simulink model "Commercial_Power_Generation_and_Transmission"  (R2022b)
settings: Solver=VariableStepAuto  StartTime=0.0  StopTime=10.0  RelTol=1e-3
libraries: spsExcitationSystemLib x6, spsHydraulicTurbineandGovernorLib x6, spsSynchronousMachinepuFundamentalLib x6, spsThreePhaseTransformerTwoWindingsLib x4, spsLoadFlowBusLib x2, spsThreePhaseParallelRLCLoadLib x2, spsGroundLib x1, spsThreePhaseFaultLib x1, spsThreePhaseSourceLib x1, spsVoltageMeasurementLib x1, spspowerguiLib x1
settings Model: Creator=admin  LastModifiedBy=USER
settings SolverCC: AlgebraicLoopSolver=TrustRegion
settings DebuggingCC: UnconnectedInputMsg=warning  UnconnectedOutputMsg=warning  UnconnectedLineMsg=warning
settings ModelReferenceCC: EnableRefExpFcnMdlSchedulingChecks=on
settings RTWCC: GenCodeOnly=on

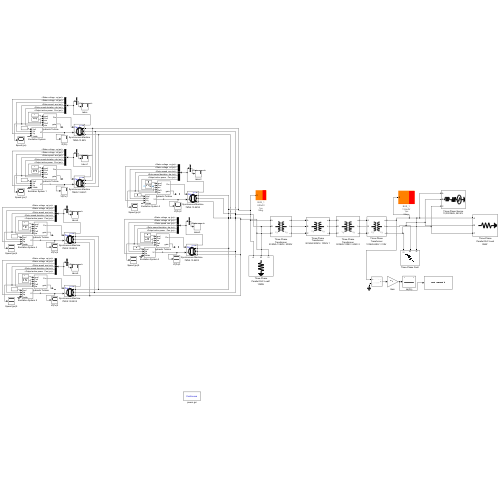
[thumbnail: Simulink's stored preview of the top-level diagram]
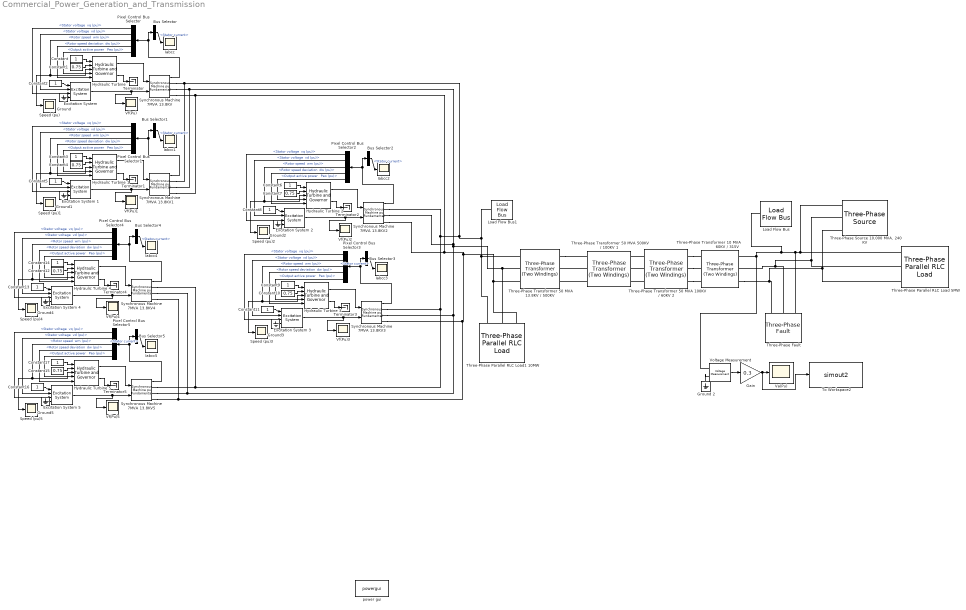
== system Commercial_Power_Generation_and_Transmission ==
  Bus Selector{,1..5} (6 alike) : BusSelector  OutputSignals=Stator current
  Constant{,2..3,5..6,8..9,11,13..14,16..17} (12 alike) : Constant
  Constant{1,4,7,10,12,15} (6 alike) : Constant  Value=0.75
  Excitation System {,1..5} (6 alike) : spsExcitationSystemLib/Excitation System  tr=20e-3  reg=[ 300, 0.001 ]  exc=[ 1, 0 ]  tgr=[ 0, 0 ]  damp=[ 0.001, 0.1 ]  sat=[ 0, 0 ]  lim=[ -11.5, 11.5, 0 ]  v0="[1.0  1.28]"
  "Gain " : Gain  Gain=0.3
  Ground{,1..5} (6 alike) : Ground
  "Ground 2 " : spsGroundLib/Ground  LConnTagsString=a
  Hydraulic Turbine {,1..5} (6 alike) : spsHydraulicTurbineandGovernorLib/Hydraulic Turbine and Governor  sm="[ 10/3  0.07 ]"  gate="[  0.01  0.97518  -0.1  0.1 ]"  reg="[  0.05  1.163  0.105  0  0.01  ]"  hyd="[  0  2.67  ]"  dref=0  po=0.7516
  Iabcc{,1..5} (6 alike) : Scope
  Load Flow Bus : spsLoadFlowBusLib/Load Flow Bus  LConnTagsString=a  Phases=single  Connectors=on one side  ID=BUS_1  Vbase=13.8e3  Vref=1  Vangle=0  VLF=1  VLFb=1  VLFc=1  angleLF=0  angleLFb=0  angleLFc=0
  Load Flow Bus1 : spsLoadFlowBusLib/Load Flow Bus  LConnTagsString=a  Phases=single  Connectors=on one side  ID=BUS_1  Vbase=240e3  Vref=1  Vangle=0  VLF=1  VLFb=1  VLFc=1  angleLF=0  angleLFb=0  angleLFc=0
  Pixel Control Bus Selector{,1..5} (6 alike) : BusSelector  OutputSignals="dq0 components.Stator voltage  vq (pu),dq0 components.Stator voltage  vd (pu),Mechanical.Rotor speed  wm (pu),Mechanical.Rotor speed deviation  dw (pu),Output active power   Peo (pu)"
  Speed (pu){,1..5} (6 alike) : Scope
  Synchronous Machine 7MVA 13.8KV{,1..5} (6 alike) : spsSynchronousMachinepuFundamentalLib/Synchronous Machine pu Fundamental  PresetModel=No  MechanicalLoad=Mechanical power Pm  ShowDetailedParameters=on  RotorType=Salient-pole  Units=per unit fundamental parameters  MeasurementBus=off  NominalParameters="[ 7E6  13800   60]"  Stator="[ 2.85E-03  0.114  1.19  0.36 ]"  Field="[ 5.79E-04  0.114]"  Dampers2=[0.0652, 0.5134, 0.0287, 0.2553, 7.765e-3, 0.9167 ]  Dampers1="[ 1.17E-02  0.182  1.97E-02  0.384 ]"  Mechanical=[ 3.7 0 20]  PolePairs=20  InitialConditions="[ 0  0  0  0  0  0  0  0  1 ]"  SetSaturation=off  Saturation=[0.6404,0.7127,0.8441,0.9214,0.9956,1.082,1.19,1.316,1.457;0.7,0.7698,0.8872,0.9466,0.9969,1.046,1.1,1.151,1.201]  LoadFlowParameters=[1,0,0,0,0]  TsPowergui=0  TsBlock=-1  IterativeModel=Trapezoidal non iterative  IterativeDiscreteModel=Trapezoidal non iterative  BusType=PV  Pref=0  Qref=0  Qmin=-inf  Qmax=inf  PLF=0  QLF=0
  Terminator{,1..5} (6 alike) : Terminator
  "Three-Phase Parallel RLC Load 5MW " : spsThreePhaseParallelRLCLoadLib/Three-Phase Parallel RLC Load  LConnTagsString=A|B|C  Configuration=Y (grounded)  NominalVoltage=13800  Vabc=[1e3 1e3 1e3]  Vabcp=[1e3 1e3 1e3]  NominalFrequency=60  UnbalancedPower=off  ActivePower=5e6  InductivePower=0  CapacitivePower=0  Pabc=[10e3 9e3 11e3]  QLabc=[100 90 110]  QCabc=[100 90 110]  Pabcp=[10e3 9e3 11e3]  QLabcp=[100 90 110]  QCabcp=[100 90 110]  Measurements=None  LoadType=constant Z
  "Three-Phase Parallel RLC Load1 10MW " : spsThreePhaseParallelRLCLoadLib/Three-Phase Parallel RLC Load  LConnTagsString=A|B|C  Configuration=Y (grounded)  NominalVoltage=240e3  Vabc=[1e3 1e3 1e3]  Vabcp=[1e3 1e3 1e3]  NominalFrequency=60  UnbalancedPower=off  ActivePower=10e6  InductivePower=0  CapacitivePower=0  Pabc=[10e3 9e3 11e3]  QLabc=[100 90 110]  QCabc=[100 90 110]  Pabcp=[10e3 9e3 11e3]  QLabcp=[100 90 110]  QCabcp=[100 90 110]  Measurements=None  LoadType=constant Z
  "Three-Phase Transformer 10 MVA 60KV / 315V " : spsThreePhaseTransformerTwoWindingsLib/Three-Phase Transformer (Two Windings)  Winding1Connection=Yg  Winding2Connection=Yg  CoreType=Three single-phase transformers  SetSaturation=off  Hysteresis=off  DataFile='hysteresis'  SetInitialFlux=off  Measurements=None  UNITS=pu  NominalPower=[ 50e6 , 60 ]  Winding1=[60e3 , 0.002 , 0.08 ]  Winding2=[315 , 0.002 , 0.08 ]  Rm=500  Lm=500  L0=0.5  Saturation=[ 0,0 ; 0.0024,1.2 ; 1.0,1.52 ]  InitialFluxes=[ 0.8 , -0.8 , 0.7 ]  BreakLoop=off  DiscreteSolver=Trapezoidal iterative  DataType=off  TransfoNumber=1
  Three-Phase Transformer 50 MVA 100KV / 60KV 2 : spsThreePhaseTransformerTwoWindingsLib/Three-Phase Transformer (Two Windings)  Winding1Connection=Yg  Winding2Connection=Yg  CoreType=Three single-phase transformers  SetSaturation=off  Hysteresis=off  DataFile='hysteresis'  SetInitialFlux=off  Measurements=None  UNITS=pu  NominalPower=[ 50e6 , 60 ]  Winding1=[ 100e3 , 0.002 , 0.08 ]  Winding2=[ 60e3 , 0.002 , 0.08 ]  Rm=500  Lm=500  L0=0.5  Saturation=[ 0,0 ; 0.0024,1.2 ; 1.0,1.52 ]  InitialFluxes=[ 0.8 , -0.8 , 0.7 ]  BreakLoop=off  DiscreteSolver=Trapezoidal iterative  DataType=off  TransfoNumber=1
  "Three-Phase Transformer 50 MVA 13.8KV / 500KV " : spsThreePhaseTransformerTwoWindingsLib/Three-Phase Transformer (Two Windings)  Winding1Connection=Yg  Winding2Connection=Yg  CoreType=Three single-phase transformers  SetSaturation=off  Hysteresis=off  DataFile='hysteresis'  SetInitialFlux=off  Measurements=None  UNITS=pu  NominalPower=[ 50e6 , 60 ]  Winding1=[ 13.8e3 , 0.002 , 0.08 ]  Winding2=[ 500e3 , 0.002 , 0.08 ]  Rm=500  Lm=500  L0=0.5  Saturation=[ 0,0 ; 0.0024,1.2 ; 1.0,1.52 ]  InitialFluxes=[ 0.8 , -0.8 , 0.7 ]  BreakLoop=off  DiscreteSolver=Trapezoidal iterative  DataType=off  TransfoNumber=1
  Three-Phase Transformer 50 MVA 500KV / 100KV 1 : spsThreePhaseTransformerTwoWindingsLib/Three-Phase Transformer (Two Windings)  Winding1Connection=Yg  Winding2Connection=Yg  CoreType=Three single-phase transformers  SetSaturation=off  Hysteresis=off  DataFile='hysteresis'  SetInitialFlux=off  Measurements=None  UNITS=pu  NominalPower=[ 50e6 , 60 ]  Winding1=[ 500e3 , 0.002 , 0.08 ]  Winding2=[ 100e3 , 0.002 , 0.08 ]  Rm=500  Lm=500  L0=0.5  Saturation=[ 0,0 ; 0.0024,1.2 ; 1.0,1.52 ]  InitialFluxes=[ 0.8 , -0.8 , 0.7 ]  BreakLoop=off  DiscreteSolver=Trapezoidal iterative  DataType=off  TransfoNumber=1
  "Three-Phase Fault " : spsThreePhaseFaultLib/Three-Phase Fault  InitialStates=0  FaultA=on  FaultB=on  FaultC=on  GroundFault=on  SwitchTimes="[0.1  0.2]"  External=off  SwitchStatus=NaN  FaultResistance=1e-3  GroundResistance=1e-3  SnubberResistance=inf  SnubberCapacitance=inf  Measurements=None
  "Three-Phase Source 10,000 MVA, 240 KV " : spsThreePhaseSourceLib/Three-Phase Source  InternalConnection=Yg  VoltagePhases=off  Voltage=(240000)*(1.00006)  PhaseAngle=-0.77547  Voltage_phases=[25e3 25e3 25e3]/sqrt(3)  PhaseAngles_phases=[0 -120 +120]  Frequency=60  NonIdealSource=on  SpecifyImpedance=on  Resistance=0.8929  Inductance=16.58e-3  ShortCircuitLevel=10000e6  BaseVoltage=240e3  XRratio=10  BusType=swing  Pref=10e3  Qref=0  Prefabc=[10e3, 10e3, 10e3]  Qrefabc=[0, 0, 0]  Qmin=-inf  Qmax=inf
  To Workspace2 : ToWorkspace  VariableName=simout2  SaveFormat=Timeseries  SampleTime=-1
  Va(Pu) : Scope
  Vf(Pu){,1..5} (6 alike) : Scope
  Voltage Measurement : spsVoltageMeasurementLib/Voltage Measurement  PhasorSimulation=off  OutputType=Complex  PSBequivalent=0
  power gui : spspowerguiLib/powergui  Priority=1  SimulationMode=Continuous  SampleTime=50e-6  frequency=60  Iterations=50  frequencyindice=60  Pbase=100e6  ErrMax=1e-4  UnitsV=kV  UnitsW=MW  buscounter=0  FunctionMessages=off  echomessages=off  EnableUseOfTLC=off  CurrentSourceSwitches=off  DisableSnubberDevices=off  DisableRonSwitches=off  DisableVfSwitches=off  DisplayEquations=off  AutomaticDiscreteSolvers=off  SolverType=Tustin/Backward Euler (TBE)  Interpol=off  ExternalGateDelay=off  methode=off  Ts=100  x0status=blocks  SPID=on  SwTol=0  HookPort=off  NonlinearTolerance=1e-4  nMaxIteration=100  ContinueOnMaxIteration=off  RestoreLinks=warning  ResistiveCurrentMeasurement=off  Frange=[0:2:500]  Ylog=off  Xlog=on  ShowGrid=off  save=off  variable=ZData  structure=0  ZoomFFT=off  StartTime=0.0  cycles=1  DisplayStyle=1  fundamental=60  FreqAxis=off  MaxFrequency=1000  frequencyindicesteady=1  RmsSteady=1  display=off
  wires:
  Constant/1 -> "Hydraulic Turbine "/1
  Constant1/1 -> "Hydraulic Turbine "/2
  Constant2/1 -> "Excitation System "/1
  Ground/1 -> "Excitation System "/4
  "Hydraulic Turbine "/2 -> Terminator/1
  "Excitation System "/1 -> Vf(Pu)/1, Synchronous Machine 7MVA 13.8KV/2
  "Hydraulic Turbine "/1 -> Synchronous Machine 7MVA 13.8KV/1
  Bus Selector/1 -> Iabcc/1  "<Stator current>"
  Pixel Control Bus Selector/1 -> "Excitation System "/3  "<Stator voltage  vq (pu)>"
  Pixel Control Bus Selector/2 -> "Excitation System "/2  "<Stator voltage  vd (pu)>"
  Pixel Control Bus Selector/4 -> "Hydraulic Turbine "/5  "<Rotor speed deviation  dw (pu)>"
  Pixel Control Bus Selector/5 -> "Hydraulic Turbine "/4  "<Output active power   Peo (pu)>"
  Pixel Control Bus Selector/3 -> "Hydraulic Turbine "/3, Speed (pu)/1  "<Rotor speed  wm (pu)>"
  Synchronous Machine 7MVA 13.8KV/1 -> Bus Selector/1, Pixel Control Bus Selector/1
  Synchronous Machine 7MVA 13.8KV1/1 -> Pixel Control Bus Selector1/1, Bus Selector1/1
  Pixel Control Bus Selector1/3 -> Speed (pu)1/1, Hydraulic Turbine 1/3  "<Rotor speed  wm (pu)>"
  Pixel Control Bus Selector1/5 -> Hydraulic Turbine 1/4  "<Output active power   Peo (pu)>"
  Pixel Control Bus Selector1/4 -> Hydraulic Turbine 1/5  "<Rotor speed deviation  dw (pu)>"
  Pixel Control Bus Selector1/2 -> Excitation System 1/2  "<Stator voltage  vd (pu)>"
  Pixel Control Bus Selector1/1 -> Excitation System 1/3  "<Stator voltage  vq (pu)>"
  Bus Selector1/1 -> Iabcc1/1  "<Stator current>"
  Hydraulic Turbine 1/1 -> Synchronous Machine 7MVA 13.8KV1/1
  Excitation System 1/1 -> Synchronous Machine 7MVA 13.8KV1/2, Vf(Pu)1/1
  Hydraulic Turbine 1/2 -> Terminator1/1
  Ground1/1 -> Excitation System 1/4
  Constant5/1 -> Excitation System 1/1
  Constant4/1 -> Hydraulic Turbine 1/2
  Constant3/1 -> Hydraulic Turbine 1/1
  Constant6/1 -> Hydraulic Turbine 2/1
  Constant7/1 -> Hydraulic Turbine 2/2
  Constant8/1 -> Excitation System 2/1
  Ground2/1 -> Excitation System 2/4
  Hydraulic Turbine 2/2 -> Terminator2/1
  Excitation System 2/1 -> Vf(Pu)2/1, Synchronous Machine 7MVA 13.8KV2/2
  Hydraulic Turbine 2/1 -> Synchronous Machine 7MVA 13.8KV2/1
  Bus Selector2/1 -> Iabcc2/1  "<Stator current>"
  Pixel Control Bus Selector2/1 -> Excitation System 2/3  "<Stator voltage  vq (pu)>"
  Pixel Control Bus Selector2/2 -> Excitation System 2/2  "<Stator voltage  vd (pu)>"
  Pixel Control Bus Selector2/4 -> Hydraulic Turbine 2/5  "<Rotor speed deviation  dw (pu)>"
  Pixel Control Bus Selector2/5 -> Hydraulic Turbine 2/4  "<Output active power   Peo (pu)>"
  Pixel Control Bus Selector2/3 -> Hydraulic Turbine 2/3, Speed (pu)2/1  "<Rotor speed  wm (pu)>"
  Synchronous Machine 7MVA 13.8KV2/1 -> Bus Selector2/1, Pixel Control Bus Selector2/1
  Synchronous Machine 7MVA 13.8KV3/1 -> Pixel Control Bus Selector3/1, Bus Selector3/1
  Pixel Control Bus Selector3/3 -> Speed (pu)3/1, Hydraulic Turbine 3/3  "<Rotor speed  wm (pu)>"
  Pixel Control Bus Selector3/5 -> Hydraulic Turbine 3/4  "<Output active power   Peo (pu)>"
  Pixel Control Bus Selector3/4 -> Hydraulic Turbine 3/5  "<Rotor speed deviation  dw (pu)>"
  Pixel Control Bus Selector3/2 -> Excitation System 3/2  "<Stator voltage  vd (pu)>"
  Pixel Control Bus Selector3/1 -> Excitation System 3/3  "<Stator voltage  vq (pu)>"
  Bus Selector3/1 -> Iabcc3/1  "<Stator current>"
  Hydraulic Turbine 3/1 -> Synchronous Machine 7MVA 13.8KV3/1
  Excitation System 3/1 -> Synchronous Machine 7MVA 13.8KV3/2, Vf(Pu)3/1
  Hydraulic Turbine 3/2 -> Terminator3/1
  Ground3/1 -> Excitation System 3/4
  Constant11/1 -> Excitation System 3/1
  Constant10/1 -> Hydraulic Turbine 3/2
  Constant9/1 -> Hydraulic Turbine 3/1
  Constant14/1 -> Hydraulic Turbine 4/1
  Constant12/1 -> Hydraulic Turbine 4/2
  Constant13/1 -> Excitation System 4/1
  Ground4/1 -> Excitation System 4/4
  Hydraulic Turbine 4/2 -> Terminator4/1
  Excitation System 4/1 -> Vf(Pu)4/1, Synchronous Machine 7MVA 13.8KV4/2
  Hydraulic Turbine 4/1 -> Synchronous Machine 7MVA 13.8KV4/1
  Bus Selector4/1 -> Iabcc4/1  "<Stator current>"
  Pixel Control Bus Selector4/1 -> Excitation System 4/3  "<Stator voltage  vq (pu)>"
  Pixel Control Bus Selector4/2 -> Excitation System 4/2  "<Stator voltage  vd (pu)>"
  Pixel Control Bus Selector4/4 -> Hydraulic Turbine 4/5  "<Rotor speed deviation  dw (pu)>"
  Pixel Control Bus Selector4/5 -> Hydraulic Turbine 4/4  "<Output active power   Peo (pu)>"
  Pixel Control Bus Selector4/3 -> Hydraulic Turbine 4/3, Speed (pu)4/1  "<Rotor speed  wm (pu)>"
  Synchronous Machine 7MVA 13.8KV4/1 -> Bus Selector4/1, Pixel Control Bus Selector4/1
  Synchronous Machine 7MVA 13.8KV5/1 -> Pixel Control Bus Selector5/1, Bus Selector5/1
  Pixel Control Bus Selector5/3 -> Speed (pu)5/1, Hydraulic Turbine 5/3  "<Rotor speed  wm (pu)>"
  Pixel Control Bus Selector5/5 -> Hydraulic Turbine 5/4  "<Output active power   Peo (pu)>"
  Pixel Control Bus Selector5/4 -> Hydraulic Turbine 5/5  "<Rotor speed deviation  dw (pu)>"
  Pixel Control Bus Selector5/2 -> Excitation System 5/2  "<Stator voltage  vd (pu)>"
  Pixel Control Bus Selector5/1 -> Excitation System 5/3  "<Stator voltage  vq (pu)>"
  Bus Selector5/1 -> Iabcc5/1  "<Stator current>"
  Hydraulic Turbine 5/1 -> Synchronous Machine 7MVA 13.8KV5/1
  Excitation System 5/1 -> Synchronous Machine 7MVA 13.8KV5/2, Vf(Pu)5/1
  Hydraulic Turbine 5/2 -> Terminator5/1
  Ground5/1 -> Excitation System 5/4
  Constant16/1 -> Excitation System 5/1
  Constant15/1 -> Hydraulic Turbine 5/2
  Constant17/1 -> Hydraulic Turbine 5/1
  Voltage Measurement/1 -> "Gain "/1
  "Gain "/1 -> To Workspace2/1, Va(Pu)/1
  connections:
  "Ground 2 "/LConn1 -- Voltage Measurement/LConn2
  Synchronous Machine 7MVA 13.8KV2/RConn1 -- Synchronous Machine 7MVA 13.8KV4/RConn1 -- Synchronous Machine 7MVA 13.8KV5/RConn1 -- Synchronous Machine 7MVA 13.8KV3/RConn1 -- Synchronous Machine 7MVA 13.8KV1/RConn1 -- Synchronous Machine 7MVA 13.8KV/RConn1 -- "Three-Phase Parallel RLC Load1 10MW "/LConn1 -- "Three-Phase Transformer 50 MVA 13.8KV / 500KV "/LConn1 -- Load Flow Bus1/LConn1
  Synchronous Machine 7MVA 13.8KV2/RConn3 -- Synchronous Machine 7MVA 13.8KV4/RConn3 -- Synchronous Machine 7MVA 13.8KV5/RConn3 -- Synchronous Machine 7MVA 13.8KV3/RConn3 -- "Three-Phase Parallel RLC Load1 10MW "/LConn3 -- "Three-Phase Transformer 50 MVA 13.8KV / 500KV "/LConn3 -- Synchronous Machine 7MVA 13.8KV1/RConn3 -- Synchronous Machine 7MVA 13.8KV/RConn3
  "Three-Phase Parallel RLC Load 5MW "/LConn1 -- "Three-Phase Source 10,000 MVA, 240 KV "/RConn1 -- Load Flow Bus/LConn1 -- Voltage Measurement/LConn1 -- "Three-Phase Transformer 10 MVA 60KV / 315V "/RConn1 -- "Three-Phase Fault "/LConn1
  "Three-Phase Parallel RLC Load 5MW "/LConn2 -- "Three-Phase Source 10,000 MVA, 240 KV "/RConn2 -- "Three-Phase Fault "/LConn2 -- "Three-Phase Transformer 10 MVA 60KV / 315V "/RConn2
  "Three-Phase Transformer 10 MVA 60KV / 315V "/RConn3 -- "Three-Phase Source 10,000 MVA, 240 KV "/RConn3 -- "Three-Phase Parallel RLC Load 5MW "/LConn3 -- "Three-Phase Fault "/LConn3
  "Three-Phase Transformer 50 MVA 13.8KV / 500KV "/RConn1 -- Three-Phase Transformer 50 MVA 500KV / 100KV 1/LConn1
  Three-Phase Transformer 50 MVA 500KV / 100KV 1/LConn2 -- "Three-Phase Transformer 50 MVA 13.8KV / 500KV "/RConn2
  Three-Phase Transformer 50 MVA 500KV / 100KV 1/LConn3 -- "Three-Phase Transformer 50 MVA 13.8KV / 500KV "/RConn3
  Three-Phase Transformer 50 MVA 100KV / 60KV 2/LConn1 -- Three-Phase Transformer 50 MVA 500KV / 100KV 1/RConn1
  Three-Phase Transformer 50 MVA 100KV / 60KV 2/LConn2 -- Three-Phase Transformer 50 MVA 500KV / 100KV 1/RConn2
  Three-Phase Transformer 50 MVA 100KV / 60KV 2/LConn3 -- Three-Phase Transformer 50 MVA 500KV / 100KV 1/RConn3
  Three-Phase Transformer 50 MVA 100KV / 60KV 2/RConn1 -- "Three-Phase Transformer 10 MVA 60KV / 315V "/LConn1
  Three-Phase Transformer 50 MVA 100KV / 60KV 2/RConn2 -- "Three-Phase Transformer 10 MVA 60KV / 315V "/LConn2
  Three-Phase Transformer 50 MVA 100KV / 60KV 2/RConn3 -- "Three-Phase Transformer 10 MVA 60KV / 315V "/LConn3
  "Three-Phase Parallel RLC Load1 10MW "/LConn2 -- Synchronous Machine 7MVA 13.8KV1/RConn2 -- Synchronous Machine 7MVA 13.8KV/RConn2 -- Synchronous Machine 7MVA 13.8KV2/RConn2 -- Synchronous Machine 7MVA 13.8KV4/RConn2 -- Synchronous Machine 7MVA 13.8KV5/RConn2 -- Synchronous Machine 7MVA 13.8KV3/RConn2 -- "Three-Phase Transformer 50 MVA 13.8KV / 500KV "/LConn2
